simulink model "Modified_Step"  (R2023a)
settings: Solver=VariableStepAuto  StartTime=0.0  StopTime=10.0  RelTol=1e-3
undefined symbols (not defined in the file): B, J, Kd, Kp, Kt, Kw, L, R
settings Model: Creator=karteek  LastModifiedBy=karteek

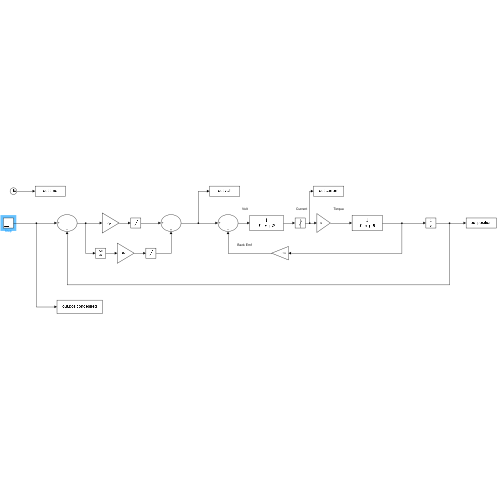
[thumbnail: Simulink's stored preview of the top-level diagram]
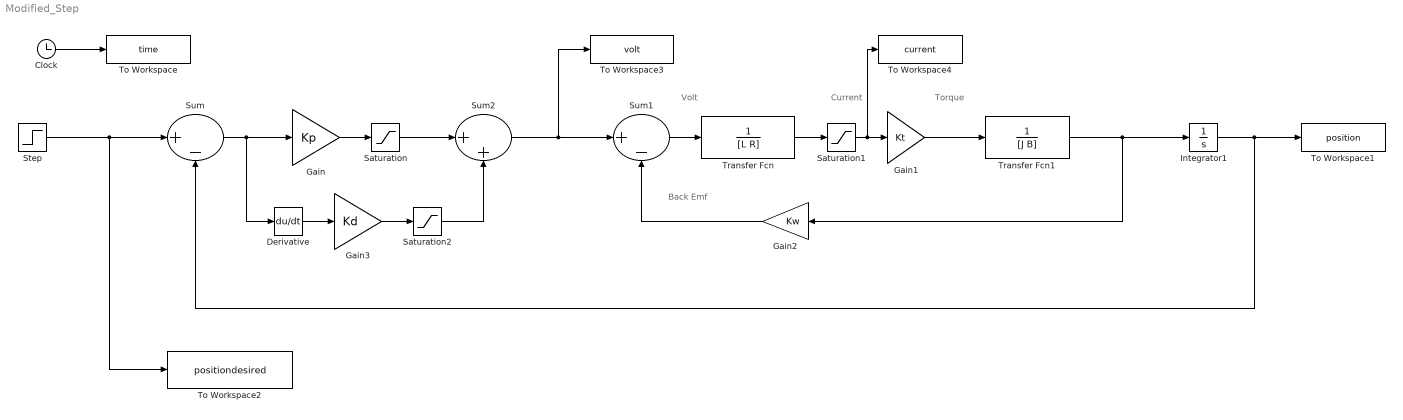
== system Modified_Step ==
  note: Volt
  note: Torque
  note: Current
  note: Back Emf
  Clock : Clock
  Derivative : Derivative
  Gain : Gain  Gain=Kp
  Gain1 : Gain  Gain=Kt
  Gain2 : Gain  Gain=Kw
  Gain3 : Gain  Gain=Kd
  Integrator1 : Integrator
  Saturation : Saturate  UpperLimit=24  LowerLimit=-24
  Saturation1 : Saturate  UpperLimit=80  LowerLimit=-80
  Saturation2 : Saturate  UpperLimit=24  LowerLimit=-24
  Step : Step  After=pi/2  SampleTime=0
  Sum : Sum  Inputs=|+-
  Sum1 : Sum  Inputs=|+-
  Sum2 : Sum  Inputs=|++
  To Workspace : ToWorkspace  VariableName=time  SampleTime=-1
  To Workspace1 : ToWorkspace  VariableName=position  SampleTime=-1
  To Workspace2 : ToWorkspace  VariableName=positiondesired  SampleTime=-1
  To Workspace3 : ToWorkspace  VariableName=volt  SampleTime=-1
  To Workspace4 : ToWorkspace  VariableName=current  SampleTime=-1
  Transfer Fcn : TransferFcn  Denominator=[L R]
  Transfer Fcn1 : TransferFcn  Denominator=[J B]
  wires:
  Sum1/1 -> Transfer Fcn/1
  Clock/1 -> To Workspace/1
  Sum/1 -> Derivative/1, Gain/1
  Gain/1 -> Saturation/1
  Transfer Fcn1/1 -> Gain2/1, Integrator1/1
  Gain2/1 -> Sum1/2
  Step/1 -> Sum/1, To Workspace2/1
  Gain1/1 -> Transfer Fcn1/1
  Transfer Fcn/1 -> Saturation1/1
  Saturation1/1 -> To Workspace4/1, Gain1/1
  Saturation/1 -> Sum2/1
  Sum2/1 -> To Workspace3/1, Sum1/1
  Derivative/1 -> Gain3/1
  Gain3/1 -> Saturation2/1
  Saturation2/1 -> Sum2/2
  Integrator1/1 -> Sum/2, To Workspace1/1
